simulink model "PGS_PDpG"  (R2017b)
settings: Solver=ode45  StartTime=0.0  StopTime=15  MaxStep=0.02  RelTol=1e-3
settings Model: Creator=Enrique Benavides  LastModifiedBy=Enrique Benavides

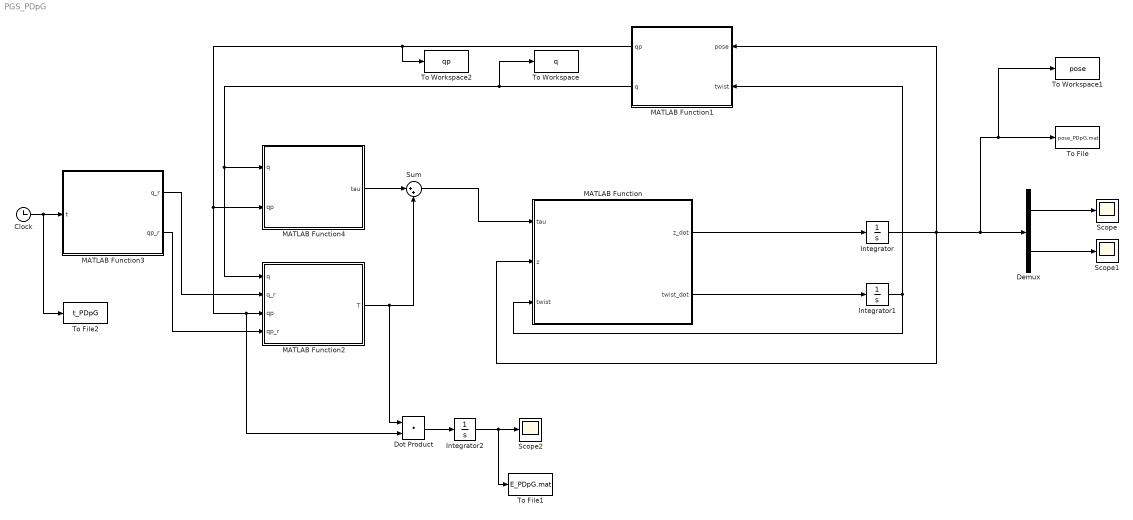
== system PGS_PDpG ==
  Clock : Clock
  Demux : Demux  Outputs=2
  Dot Product : DotProduct  InputSameDT=on  OutDataTypeStr=Inherit: Inherit via internal rule
  Integrator : Integrator  InitialCondition=[0;0;1.3;0;0;0]
  Integrator1 : Integrator  InitialCondition=[0;0;0;0;0;0]
  Integrator2 : Integrator
  MATLAB Function : MATLAB Function  TreatAsAtomicUnit=on
  MATLAB Function1 : MATLAB Function  TreatAsAtomicUnit=on
  MATLAB Function2 : MATLAB Function  TreatAsAtomicUnit=on
  MATLAB Function3 : MATLAB Function  TreatAsAtomicUnit=on
  MATLAB Function4 : MATLAB Function  TreatAsAtomicUnit=on
  Scope : Scope
  Scope1 : Scope
  Scope2 : Scope
  Sum : Sum  Inputs=|++
  To File : ToFile  Filename=pose_PDpG.mat  MatrixName=pose  SaveFormat=Timeseries
  To File1 : ToFile  Filename=E_PDpG.mat  MatrixName=en_PDpG  SaveFormat=Timeseries
  To File2 : ToFile  Filename=t_PDpG  MatrixName=tout  SaveFormat=Timeseries
  To Workspace : ToWorkspace  VariableName=q  SampleTime=-1
  To Workspace1 : ToWorkspace  VariableName=pose  SampleTime=-1
  To Workspace2 : ToWorkspace  VariableName=qp  SampleTime=-1
  wires:
  MATLAB Function/1(z_dot) -> Integrator/1
  MATLAB Function/2(twist_dot) -> Integrator1/1
  Integrator1/1 -> MATLAB Function1/2(twist), MATLAB Function/3(twist)
  Demux/1 -> Scope/1
  Demux/2 -> Scope1/1
  MATLAB Function1/1(qp) -> To Workspace2/1, MATLAB Function4/2(qp), Dot Product/2, MATLAB Function2/3(qp)
  MATLAB Function1/2(q) -> To Workspace/1, MATLAB Function4/1(q), MATLAB Function2/1(q)
  Integrator/1 -> MATLAB Function1/1(pose), To Workspace1/1, To File/1, Demux/1, MATLAB Function/2(z)
  MATLAB Function3/1(q_r) -> MATLAB Function2/2(q_r)
  MATLAB Function4/1(tau) -> Sum/1
  Sum/1 -> MATLAB Function/1(tau)
  MATLAB Function2/1(T) -> Dot Product/1, Sum/2
  Dot Product/1 -> Integrator2/1
  Integrator2/1 -> To File1/1, Scope2/1
  MATLAB Function3/2(qp_r) -> MATLAB Function2/4(qp_r)
  Clock/1 -> To File2/1, MATLAB Function3/1(t)

== matlab function PGS_PDpG/MATLAB Function1 ==
  data: qp output; pose input; q output; twist input
function [qp,q] = fcn(pose,twist)
d = pose(1:3);
R = ROT(pose(6),'z','r')*ROT(pose(5),'y','r')*ROT(pose(4),'x','r');

[anga,angb,a,b,lmin,I] = PGS_data();
l = zeros(3,6);
q = zeros(6,1);
lam = zeros(3,6);

for i = 1:6
    l(:,i) = d + R*a(:,i) - b(:,i);
    q(i)=norm(l(:,i));
    lam(:,i) = l(:,i)/q(i);
end

A = zeros(6,6);
for i = 1:6
    A(i,1:3) = lam(:,i)';
    d = R*a(:,i);
    cc = cross(d,lam(:,i));
    A(i,4:6) = cc';
end

qp = A*twist;

end

== matlab function PGS_PDpG/MATLAB Function ==
  data: tau input; z input; z_dot output; twist input; twist_dot output
function [z_dot,twist_dot] = fcn(tau,z,twist)

[anga,angb,a,b,lmin,I] = PGS_data();      % Parametros plataforma
d = z(1:3);                               % Distancia de la plataforma [x,y,z]^T
R = z(4:6);                               % Orientacion de plataforma [psi,theta,phi]^T

%% Cinemática inversa plataforma
[q,lambda] = IK(d,R,a,b);

%% pseudo-Cinemática inversa
th_i = p_IK(R,q,lambda,anga,angb);
[X_plu, J,t_dot] = p_IVK2(th_i,lambda,lmin,twist);

twist_dot = Q_LIK2(J,t_dot,X_plu,twist,lambda,tau,R,a,I);

z_dot = inv(op_cin(R))*twist;
end

== matlab function PGS_PDpG/MATLAB Function2 ==
  data: q input; T output; q_r input; qp input; qp_r input
function T = fcn(q,q_r,qp,qp_r)
eq = q_r - q;
eqp = qp_r - qp;
hii = [4.8849;4.8849;4.8849;4.8849;4.8849;4.8849]*10000;
G = [3.2719;3.2719;3.2719;3.2719;3.2719;3.2719]*1000;
w = 4;

Kp = diag(hii)*(w^2);
Kd = diag(hii)*(2*w);

T = (Kp*eq) + (Kd*eqp) + G;

end

== matlab function PGS_PDpG/MATLAB Function3 ==
  data: t input; q_r output; qp_r output
function [q_r,qp_r]  = fcn(t)
A = zeros(6,6);

% Constantes para el movimiento
w = (2*pi)/10;                 % Frecuencia de 1/5 Hz
r = .1;                       % Radio movimiento

x = r*cos(w*t);               % Posicion x
y = r*sin(w*t);               % Posicion y
z = 1.5;                      % Posicion z
ang = [0,0,0];                % Posicion angular

dx = -w*r*sin(w*t);           % Velocidad x
dy = w*r*cos(w*t);            % Velocidad y
dz = 0;                       % Velocidad z
dang = [0,0,0];               % Velocidad angular


twist = [dx,dy,dz,dang]';
d = [x,y,z]';
R = ROT(ang(3),'z','r')*ROT(ang(2),'y','r')*ROT(ang(1),'x','r');

l = zeros(3,6); q_r = zeros(6,1); lam = zeros(3,6);
[~,~,a,b,~,~] = PGS_data();

for i = 1:6
    l(:,i) = d + R*a(:,i) - b(:,i);
    q_r(i)=norm(l(:,i));
    lam(:,i) = l(:,i)/q_r(i);
end

%Jacobiano geometrico inverso
for i = 1:6
    A(i,1:3) = lam(:,i)';
    d = R*a(:,i);
    cc = cross(d,lam(:,i));
    A(i,4:6) = cc';
end

qp_r = A*twist;

end

== matlab function PGS_PDpG/MATLAB Function4 ==
  data: q input; tau output; qp input
function tau = fcn(q,qp)
tau=zeros(6,1);
Lmin=1.28929; 
Lmax=2.28929; 
Kp=2000000;
Kb=2500;
for i=1:6
    desp=q(i);
    vel=qp(i);
    if (desp < Lmin)
        tau(i)=(Kp*(Lmin-desp))-(Kb*(vel));
    elseif (desp > Lmax)
        tau(i)=(Kp*(Lmax-desp))-(Kb*(vel));
    end
end

end
